simulink model "serialtester1"  (R2018b)
settings: Solver=VariableStepAuto  StartTime=0.0  StopTime=inf  RelTol=1e-3
undefined symbols (not defined in the file or in its folder): serial
libraries: instrumentlib x3
settings Model: Creator=Robert  LastModifiedBy=Robert

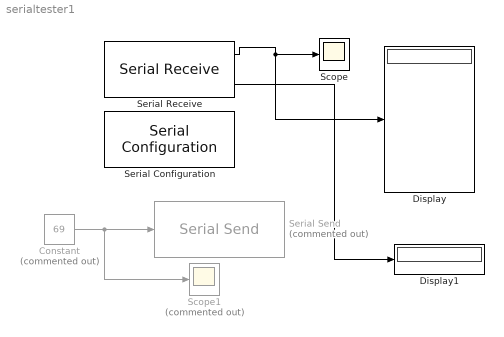
== system serialtester1 ==
  Constant : Constant  Commented=on  Value=69  OutDataTypeStr=uint8  SampleTime=0.1
  Display : Display
  Display1 : Display
  Scope : Scope
  Scope1 : Scope  Commented=on
  Serial Configuration : instrumentlib/Serial Configuration  Priority=-200000  ComPortMenu=COM12  ComPort=COM12  ObjConstructor=serial('COM12');  BaudRate=57600  DataBits=8  Parity=none  StopBits=1  FlowControl=none  Timeout=3  ByteOrder=LittleEndian
  Serial Receive : instrumentlib/Serial Receive  ComPortMenu=COM12  ComPort=COM12  ObjConstructor=serial('COM12');  Header=A  Terminator=<none>  DataSize="[2  1]"  DataType=uint8  EnableBlockingMode=off  ActionDataUnavailable=Output last received value  CustomValue=0  SampleTime=0.01
  Serial Send : instrumentlib/Serial Send  Commented=on  ComPortMenu=<Please select a port...>  ComPort=COM12  ObjConstructor=serial('COM12');  Header=A  Terminator=<none>  EnableBlockingMode=on
  wires:
  Serial Receive/1 -> Display/1, Scope/1
  Constant/1 -> Scope1/1, Serial Send/1
  Serial Receive/2 -> Display1/1
